simulink library "rw_valid_lib"  (R2018b)
settings: Solver=VariableStepAuto  StartTime=0.0  StopTime=10.0  RelTol=1e-3
undefined symbols (not defined in the file or in its folder): fsw_params
libraries: simulink x4
settings Model: Creator=taylorreynolds  LastModifiedBy=Taylor
settings SFSimCC: SimUseLocalCustomCode=off
settings RTWCC: RTWUseLocalCustomCode=off
settings CodeAppCC: StateflowObjectComments=on

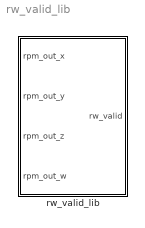
== system rw_valid_lib ==
  rw_valid_lib : Subsystem

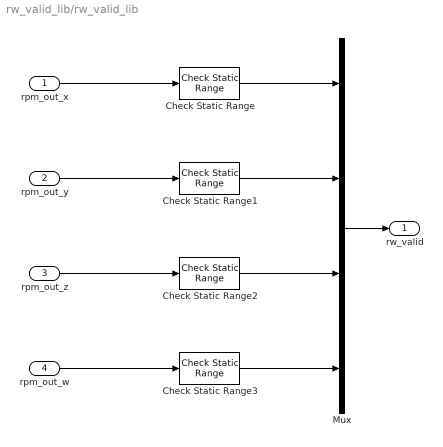
== system rw_valid_lib/rw_valid_lib ==
  rpm_out_x : Inport
  "rpm_out_y " : Inport  Port=2
  "rpm_out_z " : Inport  Port=3
  rpm_out_w : Inport  Port=4
  Check Static Range{,1..3} (4 alike) : simulink/Model Verification/Check  Static Range  Description=-fsw_params.actuators.reaction_wheel.max_RPM <= u <= fsw_params.actuators.reaction_wheel.max_RPM  max=fsw_params.actuators.reaction_wheel.max_RPM  max_included=on  min=-fsw_params.actuators.reaction_wheel.max_RPM  min_included=on  enabled=on  stopWhenAssertionFail=off  export=on  icon=graphic
      settings: SourceProductName=Simulink  SourceProductBaseCode=SL
  Mux : Mux
  rw_valid : Outport
  wires:
  rpm_out_x/1 -> Check Static Range/1
  "rpm_out_y "/1 -> Check Static Range1/1
  "rpm_out_z "/1 -> Check Static Range2/1
  Check Static Range1/1 -> Mux/2
  Check Static Range/1 -> Mux/1
  Check Static Range2/1 -> Mux/3
  Mux/1 -> rw_valid/1
  rpm_out_w/1 -> Check Static Range3/1
  Check Static Range3/1 -> Mux/4
